simulink model "hil3_host_demo"  (Simulink 7.3)
settings: Solver=ode45  StartTime=0.0  StopTime=5  RelTol=1e-3
settings Model: Creator=Krisada  LastModifiedBy=Krisada

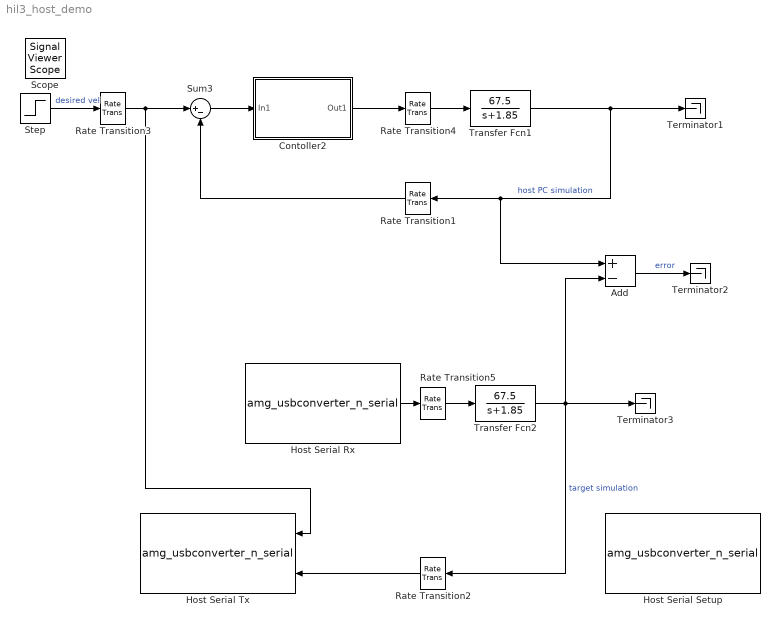
== system hil3_host_demo ==
  Add : Sum  Inputs=+-  OutDataType=fixdt(1, 16)  OutScaling=2^-10
  Contoller2 : Subsystem
  Host Serial Rx : S-Function  Priority=1  FunctionName=amg_usbconverter_n_serial  Parameters=configuration,port,transfer,baudrate,stopbit,inputtype,outputtype,binheaderarray,binterminatorarray,asciiheader,asciiterminator,bindatalength,packetmode,timeout,sampletime,initialvalues,blockid  EnableBusSupport=off  mask(amg_usbconverter_n_serial){configuration=Rx, port=COM22, baudrate=115200, databits=8, parity=None, stopbit=1, flowcontrol=None, advanceoptions=off, rxbuffersize=2048, txbuffersize=2048, transfer=Blocking, enableinitial=off, initialvalues=[], timeout=5, packetmode=Binary, binheader='7E 7E', binterminator='03 03', porttype_double=1, porttype_single=0, porttype_int8=0, porttype_uint8=0, porttype_int16=0, porttype_uint16=0, porttype_int32=0, porttype_uint32=0, asciiformat='%d,%f', rx_asciiterminator=LF (0x0A - "\n"), tx_asciiterminator=LF (0x0A - "\n"), inputtype=[0], outputtype=[1  0], binheaderarray=[2 126  126], binterminatorarray=[2 3  3], bindatalength=8, asciiheader=['%d,%f' uint8(10)], asciiterminator=[1 10], sampletime=0.005, sampletimestr=, blockid=HostSerialRx}
      mask prompts: baudrate "Baud rate (bps)"; databits "Data bits"; stopbit "Stop bit"; flowcontrol "Hardware flow control"; advanceoptions "Advance options"; rxbuffersize "Rx buffer size (bytes)"; txbuffersize "Tx buffer size (bytes)"; enableinitial "Enable initial value  (Closed loop HIL test)"; initialvalues "Initial values"; timeout "Wait time-out (Seconds)"; packetmode "Packet mode"; binheader "Binary header (example: '7E 7E')"; binterminator "Binary terminator (example: '03 03')"; porttype_double "Number of data port, type DOUBLE"; porttype_single "Number of data port, type SINGLE"; porttype_int8 "Number of data port, type INT8"; porttype_uint8 "Number of data port, type UINT8"; porttype_int16 "Number of data port, type INT16"; porttype_uint16 "Number of data port, type UINT16"; porttype_int32 "Number of data port, type INT32"; porttype_uint32 "Number of data port, type UINT32"; asciiformat "Ascii format"; rx_asciiterminator "End of packet"; tx_asciiterminator "End of packet"; inputtype "Input data type"; outputtype "Output data type"; binheaderarray "Binary header"; binterminatorarray "Binary terminator"; bindatalength "Binary data length"; asciiheader "Ascii header (printf format)"; asciiterminator "Ascii terminator"; sampletime "Sample time (sec)"; sampletimestr "Compiled sample time (sec) in string"
      mask help:
      | Enable initial value (Closed loop HIL test):
      |  - Checked: The block will return a initial value (constant) at first time step.
      |  - Unchecked: Normal operation, the block waiting for matched packet data before return value.
      mask init:
      | amg_usbconverter_n_serial_callback('init');
      mask Help: web(fullfile(waijungdocroot,'amg_usbconverter_n_uart.htm'), '-browser')
      mask StyleString: popup(Setup|Tx|Rx),popup(COM3|COM22|COM23),edit,popup(8),popup(None),popup(1|1.5|2),popup(None|RTS|CTS|RTS/CTS),checkbox,popup(16|32|64|128|256|512|1024|2048),popup(16|32|64|128|256|512|1024|2048),popup(Blocking|Non-Blocking),checkbox,edit,edit,popup(Ascii|Binary),edit,edit,edit,edit,edit,edit,edit,edit,edit,edit,edit,popup(CR (0x0D - "\r")|LF (0x0A - "\n")|CRLF (0x0D 0x0A - "\r\n")),popup(CR (0x0D - "\r")|LF (0x0A - "\n")|CRLF (0x0D 0x0A - "\r\n")|None),edit,edit,edit,edit,edit,edit,edit,edit,edit,edit
      mask CallbackString: amg_usbconverter_n_serial_callback('configuration');|amg_usbconverter_n_serial_callback('port');|amg_usbconverter_n_serial_callback('baudrate');||||amg_usbconverter_n_serial_callback('flowcontrol');|amg_usbconverter_n_serial_callback('advanceoptions');|||amg_usbconverter_n_serial_callback('transfer');|amg_usbconverter_n_serial_callback('enableinitial');|amg_usbconverter_n_serial_callback('initialvalues');||amg_usbconverter_n_serial_callback('packetmode');|amg_usbconverter_n_serial_callback('binheader');|amg_usbconverter_n_serial_callback('binterminator');|amg_usbconverter_n_serial_callback('porttype');|amg_usbconverter_n_serial_callback('porttype');|amg_usbconverter_n_serial_callback('porttype');|amg_usbconverter_n_serial_callback('porttype');|amg_usbconverter_n_serial_callback('porttype');|amg_usbconverter_n_serial_callback('porttype');|amg_usbconverter_n_serial_callback('porttype');|amg_usbconverter_n_serial_callback('porttype');|amg_usbconverter_n_serial_callback('asciiformat');|amg_usbconverter_n_serial_callback('rx_asciiterminator');|amg_usbconverter_n_serial_callback('tx_asciiterminator');||||||||amg_usbconverter_n_serial_callback('sampletime');|amg_usbconverter_n_serial_callback('sampletimestr');|amg_usbconverter_n_serial_callback('blockid');
      mask Display: text(0.05, 0.5, 'Port: COM22\nPacket: Binary\nTransfer: Blocking\nTs (sec): 0.005','ver','middle','hor','left');port_label('output', 1,'double');
  Host Serial Setup : S-Function  Priority=1  FunctionName=amg_usbconverter_n_serial  Parameters=configuration,port,transfer,baudrate,stopbit,inputtype,outputtype,binheaderarray,binterminatorarray,asciiheader,asciiterminator,bindatalength,packetmode,timeout,sampletime,sampletimestr,blockid  EnableBusSupport=off  mask(amg_usbconverter_n_serial){configuration=Setup, port=COM22, baudrate=115200, databits=8, parity=None, stopbit=1, flowcontrol=None, advanceoptions=off, rxbuffersize=2048, txbuffersize=2048, transfer=Blocking, timeout=5, packetmode=Binary, binheader='7E 7E', binterminator='03 03', porttype_double=1, porttype_single=0, porttype_int8=1, porttype_uint8=0, porttype_int16=0, porttype_uint16=0, porttype_int32=0, porttype_uint32=0, asciiformat='%d,%f', rx_asciiterminator=CRLF (0x0D 0x0A - "\r\n"), tx_asciiterminator=CR (0x0D - "\r"), inputtype=[0], outputtype=[0], binheaderarray=[2 126  126], binterminatorarray=[2 3  3], bindatalength=0, asciiheader='', asciiterminator=[0], sampletime=inf, sampletimestr=, blockid=HostSerialSetup}
      mask prompts: baudrate "Baud rate (bps)"; databits "Data bits"; stopbit "Stop bit"; flowcontrol "Hardware flow control"; advanceoptions "Advance options"; rxbuffersize "Rx buffer size (bytes)"; txbuffersize "Tx buffer size (bytes)"; timeout "Wait time-out (Seconds)"; packetmode "Packet mode"; binheader "Binary header (example: '7E 7E')"; binterminator "Binary terminator (example: '03 03')"; porttype_double "Number of data port, type DOUBLE"; porttype_single "Number of data port, type SINGLE"; porttype_int8 "Number of data port, type INT8"; porttype_uint8 "Number of data port, type UINT8"; porttype_int16 "Number of data port, type INT16"; porttype_uint16 "Number of data port, type UINT16"; porttype_int32 "Number of data port, type INT32"; porttype_uint32 "Number of data port, type UINT32"; asciiformat "Ascii format"; rx_asciiterminator "End of packet"; tx_asciiterminator "End of packet"; inputtype "Input data type"; outputtype "Output data type"; binheaderarray "Binary header"; binterminatorarray "Binary terminator"; bindatalength "Binary data length"; asciiheader "Ascii header (printf format)"; asciiterminator "Ascii terminator"; sampletime "Sample time (sec)"; sampletimestr "Compiled sample time (sec) in string"
      mask init:
      | amg_usbconverter_n_serial_callback('init');
      mask Help: web(fullfile(waijungdocroot,'amg_usbconverter_n_uart.htm'), '-browser')
      mask StyleString: popup(Setup|Tx|Rx),popup(COM3|COM22|COM23),edit,popup(8),popup(None),popup(1|1.5|2),popup(None|RTS|CTS|RTS/CTS),checkbox,popup(16|32|64|128|256|512|1024|2048),popup(16|32|64|128|256|512|1024|2048),popup(Blocking|Non-Blocking),edit,popup(Ascii|Binary),edit,edit,edit,edit,edit,edit,edit,edit,edit,edit,edit,popup(CR (0x0D - "\r")|LF (0x0A - "\n")|CRLF (0x0D 0x0A - "\r\n")),popup(CR (0x0D - "\r")|LF (0x0A - "\n")|CRLF (0x0D 0x0A - "\r\n")|None),edit,edit,edit,edit,edit,edit,edit,edit,edit,edit
      mask CallbackString: amg_usbconverter_n_serial_callback('configuration');|amg_usbconverter_n_serial_callback('port');|amg_usbconverter_n_serial_callback('baudrate');||||amg_usbconverter_n_serial_callback('flowcontrol');|amg_usbconverter_n_serial_callback('advanceoptions');|||amg_usbconverter_n_serial_callback('transfer');||amg_usbconverter_n_serial_callback('packetmode');|amg_usbconverter_n_serial_callback('binheader');|amg_usbconverter_n_serial_callback('binterminator');|amg_usbconverter_n_serial_callback('porttype');|amg_usbconverter_n_serial_callback('porttype');|amg_usbconverter_n_serial_callback('porttype');|amg_usbconverter_n_serial_callback('porttype');|amg_usbconverter_n_serial_callback('porttype');|amg_usbconverter_n_serial_callback('porttype');|amg_usbconverter_n_serial_callback('porttype');|amg_usbconverter_n_serial_callback('porttype');|amg_usbconverter_n_serial_callback('asciiformat');|amg_usbconverter_n_serial_callback('rx_asciiterminator');|amg_usbconverter_n_serial_callback('tx_asciiterminator');||||||||amg_usbconverter_n_serial_callback('sampletime');|amg_usbconverter_n_serial_callback('sampletimestr');|amg_usbconverter_n_serial_callback('blockid');
      mask Display: text(0.5, 0.5, 'Port: COM22\nBaud (Bps): 115200\nFrame: 8-None-1','ver','middle','hor','center');
  Host Serial Tx : S-Function  Priority=1  FunctionName=amg_usbconverter_n_serial  Parameters=configuration,port,transfer,baudrate,stopbit,inputtype,outputtype,binheaderarray,binterminatorarray,asciiheader,asciiterminator,bindatalength,packetmode,timeout,sampletime,sampletimestr,blockid  EnableBusSupport=off  mask(amg_usbconverter_n_serial){configuration=Tx, port=COM22, baudrate=115200, databits=8, parity=None, stopbit=1, flowcontrol=None, advanceoptions=off, rxbuffersize=2048, txbuffersize=2048, transfer=Blocking, timeout=5, packetmode=Binary, binheader='7E 7E', binterminator='03 03', porttype_double=2, porttype_single=0, porttype_int8=0, porttype_uint8=0, porttype_int16=0, porttype_uint16=0, porttype_int32=0, porttype_uint32=0, asciiformat='%d,%f', rx_asciiterminator=CRLF (0x0D 0x0A - "\r\n"), tx_asciiterminator=LF (0x0A - "\n"), inputtype=[2  0 0], outputtype=[0], binheaderarray=[2 126  126], binterminatorarray=[2 3  3], bindatalength=16, asciiheader=['%d,%f' uint8(10)], asciiterminator=[1 10], sampletime=.005, sampletimestr=, blockid=HostSerialTx}
      mask prompts: baudrate "Baud rate (bps)"; databits "Data bits"; stopbit "Stop bit"; flowcontrol "Hardware flow control"; advanceoptions "Advance options"; rxbuffersize "Rx buffer size (bytes)"; txbuffersize "Tx buffer size (bytes)"; timeout "Wait time-out (Seconds)"; packetmode "Packet mode"; binheader "Binary header (example: '7E 7E')"; binterminator "Binary terminator (example: '03 03')"; porttype_double "Number of data port, type DOUBLE"; porttype_single "Number of data port, type SINGLE"; porttype_int8 "Number of data port, type INT8"; porttype_uint8 "Number of data port, type UINT8"; porttype_int16 "Number of data port, type INT16"; porttype_uint16 "Number of data port, type UINT16"; porttype_int32 "Number of data port, type INT32"; porttype_uint32 "Number of data port, type UINT32"; asciiformat "Ascii format"; rx_asciiterminator "End of packet"; tx_asciiterminator "End of packet"; inputtype "Input data type"; outputtype "Output data type"; binheaderarray "Binary header"; binterminatorarray "Binary terminator"; bindatalength "Binary data length"; asciiheader "Ascii header (printf format)"; asciiterminator "Ascii terminator"; sampletime "Sample time (sec)"; sampletimestr "Compiled sample time (sec) in string"
      mask init:
      | amg_usbconverter_n_serial_callback('init');
      mask Help: web(fullfile(waijungdocroot,'amg_usbconverter_n_uart.htm'), '-browser')
      mask StyleString: popup(Setup|Tx|Rx),popup(COM3|COM22|COM23),edit,popup(8),popup(None),popup(1|1.5|2),popup(None|RTS|CTS|RTS/CTS),checkbox,popup(16|32|64|128|256|512|1024|2048),popup(16|32|64|128|256|512|1024|2048),popup(Blocking|Non-Blocking),edit,popup(Ascii|Binary),edit,edit,edit,edit,edit,edit,edit,edit,edit,edit,edit,popup(CR (0x0D - "\r")|LF (0x0A - "\n")|CRLF (0x0D 0x0A - "\r\n")),popup(CR (0x0D - "\r")|LF (0x0A - "\n")|CRLF (0x0D 0x0A - "\r\n")|None),edit,edit,edit,edit,edit,edit,edit,edit,edit,edit
      mask CallbackString: amg_usbconverter_n_serial_callback('configuration');|amg_usbconverter_n_serial_callback('port');|amg_usbconverter_n_serial_callback('baudrate');||||amg_usbconverter_n_serial_callback('flowcontrol');|amg_usbconverter_n_serial_callback('advanceoptions');|||amg_usbconverter_n_serial_callback('transfer');||amg_usbconverter_n_serial_callback('packetmode');|amg_usbconverter_n_serial_callback('binheader');|amg_usbconverter_n_serial_callback('binterminator');|amg_usbconverter_n_serial_callback('porttype');|amg_usbconverter_n_serial_callback('porttype');|amg_usbconverter_n_serial_callback('porttype');|amg_usbconverter_n_serial_callback('porttype');|amg_usbconverter_n_serial_callback('porttype');|amg_usbconverter_n_serial_callback('porttype');|amg_usbconverter_n_serial_callback('porttype');|amg_usbconverter_n_serial_callback('porttype');|amg_usbconverter_n_serial_callback('asciiformat');|amg_usbconverter_n_serial_callback('rx_asciiterminator');|amg_usbconverter_n_serial_callback('tx_asciiterminator');||||||||amg_usbconverter_n_serial_callback('sampletime');|amg_usbconverter_n_serial_callback('sampletimestr');|amg_usbconverter_n_serial_callback('blockid');
      mask Display: text(0.05, 0.5, 'Port: COM22\nPacket: Binary\nTransfer: Blocking\nTs (sec): 0.005','ver','middle','hor','left');port_label('input', 1,'double');port_label('input', 2,'double');
  Rate Transition{1..5} (5 alike) : RateTransition  OutPortSampleTime=0.005
  Step : Step  After=700  SampleTime=0
  Sum3 : Sum  Inputs=|+-  OutDataType=fixdt(1, 16)  OutScaling=2^0
  Terminator1 : Terminator
  Terminator2 : Terminator
  Terminator3 : Terminator
  Transfer Fcn1 : TransferFcn  Numerator=67.5  Denominator=[1 1.85]
  Transfer Fcn2 : TransferFcn  Numerator=67.5  Denominator=[1 1.85]
  Scope : SignalViewerScope  IOType=viewer  NumInputPorts=2  LegendLocations="548.3333      659.6667           144      51.66667 628.3333           368            79      20.33333"  RefreshTime=0.035000
      settings: ShowLegends=on  YMin=0~-35  YMax=800~15
  wires:
  Step/1 -> Rate Transition3/1  "desired vel"
  Rate Transition3/1 -> Sum3/1, Host Serial Tx/1
  Transfer Fcn1/1 -> Terminator1/1, Rate Transition1/1, Add/1  "host PC simulation"
  Sum3/1 -> Contoller2/1(In1)
  Contoller2/1(Out1) -> Rate Transition4/1
  Rate Transition1/1 -> Sum3/2
  Add/1 -> Terminator2/1  "error"
  Transfer Fcn2/1 -> Terminator3/1, Add/2, Rate Transition2/1  "target simulation"
  Rate Transition2/1 -> Host Serial Tx/2
  Host Serial Rx/1 -> Rate Transition5/1
  Rate Transition4/1 -> Transfer Fcn1/1
  Rate Transition5/1 -> Transfer Fcn2/1

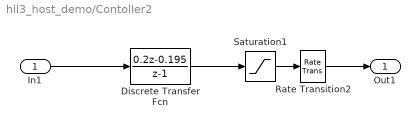
== system hil3_host_demo/Contoller2 ==
  In1 : Inport
  Discrete Transfer Fcn : DiscreteTransferFcn  Numerator=[0.2 -0.195]  Denominator=[1 -1]  SampleTime=-1
  Rate Transition2 : RateTransition
  Saturation1 : Saturate  UpperLimit=100  LowerLimit=-100  LinearizeAsGain=off  ZeroCross=off  OutDataType=fixdt(1, 16)  OutScaling=2^0
  Out1 : Outport
  wires:
  Discrete Transfer Fcn/1 -> Saturation1/1
  In1/1 -> Discrete Transfer Fcn/1
  Saturation1/1 -> Rate Transition2/1
  Rate Transition2/1 -> Out1/1
